simulink model "first"  (R2023b)
settings: Solver=VariableStepAuto  StartTime=0.0  StopTime=10.0  RelTol=1e-3
settings Model: Creator=Егор  LastModifiedBy=Егор

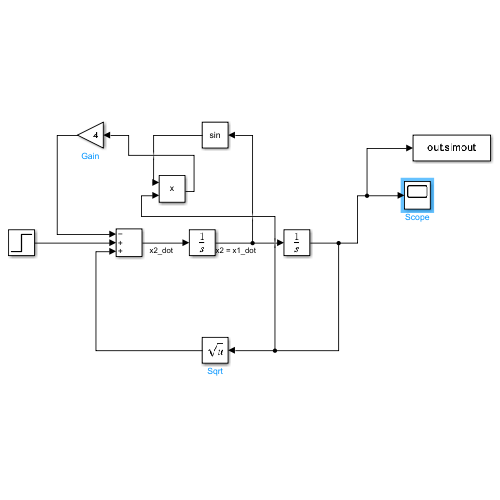
[thumbnail: Simulink's stored preview of the top-level diagram]
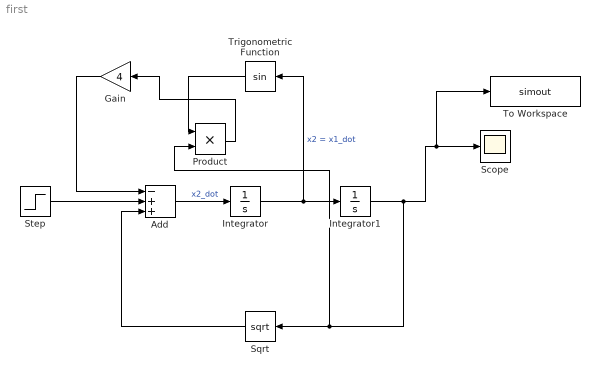
== system first ==
  Add : Sum  Inputs=-++
  Gain : Gain  Gain=4
  Integrator : Integrator
  Integrator1 : Integrator
  Product : Product
  Scope : Scope
  Sqrt : Sqrt
  Step : Step  After=0.5  SampleTime=0
  To Workspace : ToWorkspace  VariableName=simout  SampleTime=-1
  Trigonometric Function : Trigonometry
  wires:
  Step/1 -> Add/2
  Add/1 -> Integrator/1  "x2_dot"
  Integrator/1 -> Trigonometric Function/1, Integrator1/1  "x2 = x1_dot"
  Integrator1/1 -> Product/2, Sqrt/1, To Workspace/1, Scope/1
  Sqrt/1 -> Add/3
  Trigonometric Function/1 -> Product/1
  Gain/1 -> Add/1
  Product/1 -> Gain/1
